simulink model "thrAttachPtKinematics_th"  (R2018b)
settings: Solver=VariableStepAuto  StartTime=0.0  StopTime=0  RelTol=1e-3
values from neighbouring files (symbols this model uses):
  angVel = [0 0 1]    [thrAttachPtKinematics_ts.m]
libraries: thrAttachPtKinematics_ul x1
settings Model: Creator=mcobb  LastModifiedBy=mcobb

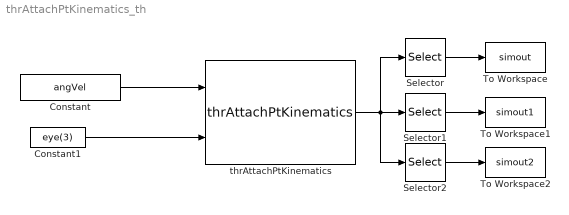
== system thrAttachPtKinematics_th ==
  Constant : Constant  Value=angVel
  Constant1 : Constant  Value=eye(3)
  Selector : Selector  InputPortWidth=3  IndexOptions=Index vector (dialog)  Indices=1  OutputSizes=1
  Selector1 : Selector  InputPortWidth=3  IndexOptions=Index vector (dialog)  Indices=1  OutputSizes=1
  Selector2 : Selector  InputPortWidth=3  IndexOptions=Index vector (dialog)  Indices=1  OutputSizes=1
  To Workspace : ToWorkspace  VariableName=simout  SaveFormat=Timeseries  SampleTime=-1
  To Workspace1 : ToWorkspace  VariableName=simout1  SaveFormat=Timeseries  SampleTime=-1
  To Workspace2 : ToWorkspace  VariableName=simout2  SaveFormat=Timeseries  SampleTime=-1
  thrAttachPtKinematics : thrAttachPtKinematics_ul/thrAttachPtKinematics  atchPts=gndStnMmtArms
  wires:
  Constant/1 -> thrAttachPtKinematics/1
  Constant1/1 -> thrAttachPtKinematics/2
  thrAttachPtKinematics/1 -> Selector1/1, Selector2/1, Selector/1
  Selector/1 -> To Workspace/1
  Selector1/1 -> To Workspace1/1
  Selector2/1 -> To Workspace2/1
